simulink model "prblm1"  (R2020b)
settings: Solver=VariableStepAuto  StartTime=0.0  StopTime=10.0  RelTol=1e-3
undefined symbols (not defined in the file): b, k1, k12, m1, m2
settings Model: Creator=shridhar  LastModifiedBy=shridhar

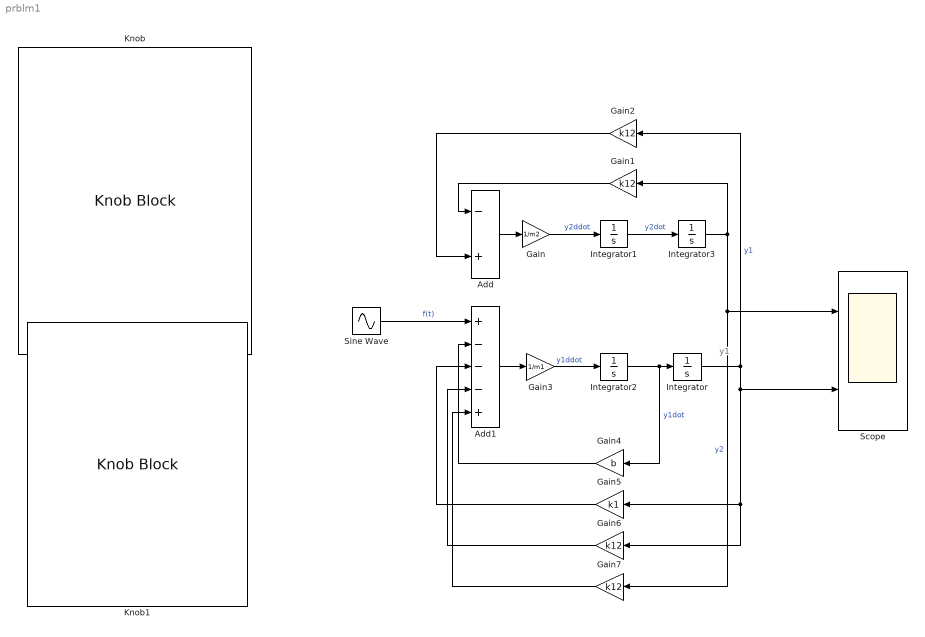
== system prblm1 ==
  note: y1
  Add : Sum  Inputs=-+
  Add1 : Sum  Inputs=+---+
  Gain : Gain  Gain=1/m2
  Gain1 : Gain  Gain=k12  ParamMin=-500  ParamMax=10000
  Gain2 : Gain  Gain=k12
  Gain3 : Gain  Gain=1/m1
  Gain4 : Gain  Gain=b
  Gain5 : Gain  Gain=k1
  Gain6 : Gain  Gain=k12
  Gain7 : Gain  Gain=k12
  Integrator : Integrator
  Integrator1 : Integrator  InitialCondition=1  IgnoreLimit=on
  Integrator2 : Integrator
  Integrator3 : Integrator
  Knob : KnobBlock  ScaleMin=-500  ScaleMax=10000
  Knob1 : KnobBlock
  Scope : Scope  NumInputPorts=2
  Sine Wave : Sin  Amplitude=2  Frequency=10  SampleTime=0
  wires:
  Gain1/1 -> Add/1
  Sine Wave/1 -> Add1/1  "f(t)"
  Gain7/1 -> Add1/5
  Gain5/1 -> Add1/3
  Gain4/1 -> Add1/2
  Gain3/1 -> Integrator2/1  "y1ddot"
  Add1/1 -> Gain3/1
  Gain/1 -> Integrator1/1  "y2ddot"
  Integrator/1 -> Scope/2, Gain6/1, Gain5/1, Gain2/1  "y1"
  Gain6/1 -> Add1/4
  Add/1 -> Gain/1
  Integrator2/1 -> Gain4/1, Integrator/1  "y1dot"
  Integrator1/1 -> Integrator3/1  "y2dot"
  Gain2/1 -> Add/2
  Integrator3/1 -> Gain7/1, Scope/1, Gain1/1  "y2"
